simulink model "subsystem_118_bus_self_clearing_blocking"  (R2025b)
settings: Solver=ode45  StartTime=0.0  StopTime=Tstop  FixedStep=Ts  RelTol=1e-12  AbsTol=1e-12
values from neighbouring files (symbols this model uses):
  gfl3_enable_before = ones(numberOfGFLs,1)    [plotFun.m]
  gfl3_enable_blocked = gfl3_enable_before    [plotFun.m]
  gfl3_enable_clear_increment = gfl3_enable_before - gfl3_enable_blocked    [plotFun.m]
  gfl3_enable_zero = zeros(numberOfGFLs,1)    [plotFun.m]
  Imax = 15    [config_file.m]
  nominalInter =     [nominalInter.mat]
  nominalU =     [nominalU.mat]
  nominalY =     [nominalY.mat]
  P_input = 0    [main_sub_118_bus.m]    (also in plotFun.m = 0.03)
  sub = struct    [main_sub_118_bus.m]
  sys_j = sys_j(1:end-1)    [IBR_modelGenerator.m]
  sys_j_AA = sys_j    [modularMOR_main.m]
  sys_j_BT = sys_j    [modularMOR_main.m]
  Tclear_gfl = 0.11    [plotFun.m]
  Tstep_gfl = 0.1    [main_sub_118_bus.m]
  Tstep_gfm = 0.1    [main_sub_118_bus.m]
  Ttrip_gfl = 0.1    [plotFun.m]
  w = 2*pi*50    (= 314.159265359)    [config_file.m]    (also in mirrorMimoWeightedFrequencyData.m = w(:); modularMOR_main.m = w(:).'; plotTest.m = w(:).')
undefined symbols (not defined in the file or in its folder): con_sub, linSys1, linSys2, linSys3
libraries: simulink x10
(part 5 of 7)

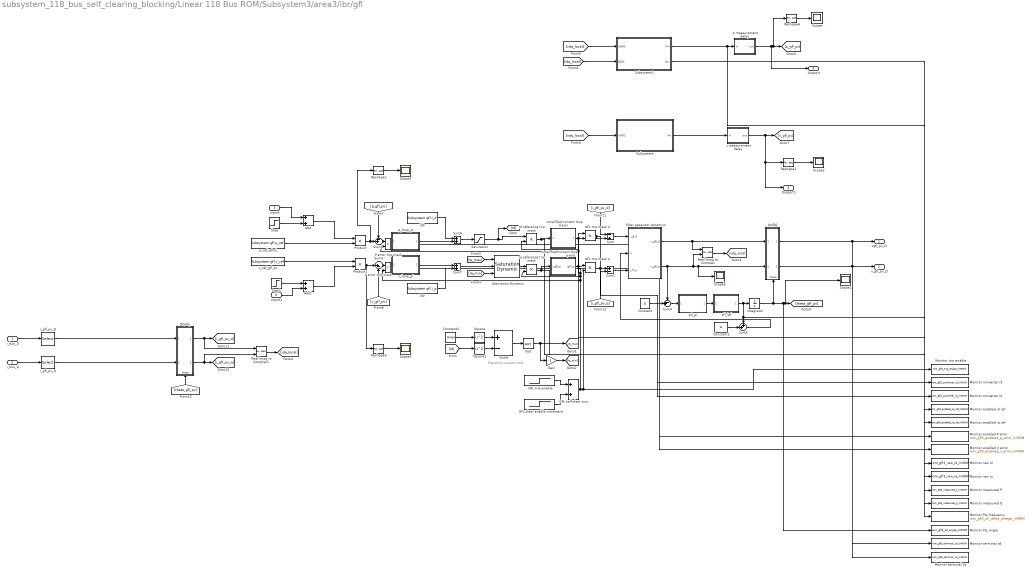
== system subsystem_118_bus_self_clearing_blocking/Linear 118 Bus ROM/Subsystem3/area3/ibr/gfl ==
  note: P-priority current limit
  i_bus_D : Inport
  i_bus_Q : Inport  Port=2
  Inport : Inport  Port=3
  Inport1 : Inport  Port=4
  Add : Sum
  Add1 : Sum
  Constant : Constant  Value=0
  Constant1 : Constant  Value=w
  Constant2 : Constant  Value=Imax
  DQ/dq : Subsystem
      settings: PortSchema="{\"entries\":[{\"content\":{\"sides\":[{\"content\":{\"connectorIds\":[\"In1\",\"In2\"]},\"type\":\"ConnectorPlacement.EquallySpacedRectSide\",\"uuid\":\"6aba5a73-e9d3-440a-9da8-5b4060b79a22\"},{\"content\":{\"connectorIds\":[\"Out1\",\"Out2\"],\"side\":\"RIGHT\"},\"type\":\"ConnectorPlacement.EquallySpacedRectSide\",\"uuid\":\"fb100e33-0f2b-446b-b234-6a01cff1cf94\"},{\"content\":{\"connectorIds\":[],\"side\":\"TOP\"},\"type\":\"ConnectorPlacement.EquallySpacedRectSide\",\"uuid\":\"cb346bab-8363-4920-b8bd-1af08716b150\"},{\"content\":{\"connectorIds\":[\"In3\"],\"side\":\"BOTTOM\"},\"type\":\"ConnectorPlacement.EquallySpacedRectSide\",\"uuid\":\"daf67601-a33f-44c6-bbbf-d32eadf086e5\"},{\"content\":{\"connectorIds\":[],\"side\":\"HIDDEN\"},\"type\":\"ConnectorPlacement.EquallySpacedRectSide\",\"uuid\":\"157b31a2-d1ec-4854-8b21-1495795af5ef\"}]},\"type\":\"ConnectorPlacement.EquallySpacedConnector\",\"uuid\":\"bdcd0df2-60ef-4202-9e13-560935cf5e64\"}],\"packageUris\":[\"http://schema.mathworks.com/mf0/Connector/R2020b\"],\"version\":\"1.0\"}"
      mask Display: image('$imagefile'); % Use "Edit Image" on toolstrip to change.
  GFL clear enable increment : Step  Time=Tclear_gfl  Before=gfl3_enable_zero  After=gfl3_enable_clear_increment  SampleTime=0
  GFL self-clear sum : Sum
  GFL trip enable : Step  Time=Ttrip_gfl  Before=gfl3_enable_before  After=gfl3_enable_blocked  SampleTime=0
  GFL trip mask d : Product  Inputs=**
  GFL trip mask q : Product  Inputs=**
  Gain : Gain  Gain=-1
  Id reference trip mask : Product  Inputs=**
  Integrator : Integrator  InitialCondition=Subsystem.gfl.theta  ContinuousStateAttributes='gfl_osc'
  Iq reference trip mask : Product  Inputs=**
  Monitor PLL angle : ToWorkspace  VariableName=rom_gfl3_pll_angle_linROM  SaveFormat=Timeseries  SampleTime=-1
  Monitor PLL frequency : ToWorkspace  VariableName=rom_gfl3_pll_delta_omega_linROM  SaveFormat=Timeseries  SampleTime=-1
  Monitor converter id : ToWorkspace  VariableName=rom_gfl3_converter_id_linROM  SaveFormat=Timeseries  SampleTime=-1
  Monitor converter iq : ToWorkspace  VariableName=rom_gfl3_converter_iq_linROM  SaveFormat=Timeseries  SampleTime=-1
  Monitor enabled P error : ToWorkspace  VariableName=rom_gfl3_enabled_p_error_linROM  SaveFormat=Timeseries  SampleTime=-1
  Monitor enabled V error : ToWorkspace  VariableName=rom_gfl3_enabled_v_error_linROM  SaveFormat=Timeseries  SampleTime=-1
  Monitor enabled id ref : ToWorkspace  VariableName=rom_gfl3_enabled_id_ref_linROM  SaveFormat=Timeseries  SampleTime=-1
  Monitor enabled iq ref : ToWorkspace  VariableName=rom_gfl3_enabled_iq_ref_linROM  SaveFormat=Timeseries  SampleTime=-1
  Monitor measured P : ToWorkspace  VariableName=rom_gfl3_measured_p_linROM  SaveFormat=Timeseries  SampleTime=-1
  Monitor measured Q : ToWorkspace  VariableName=rom_gfl3_measured_q_linROM  SaveFormat=Timeseries  SampleTime=-1
  Monitor raw id : ToWorkspace  VariableName=rom_gfl3_raw_id_linROM  SaveFormat=Timeseries  SampleTime=-1
  Monitor raw iq : ToWorkspace  VariableName=rom_gfl3_raw_iq_linROM  SaveFormat=Timeseries  SampleTime=-1
  Monitor terminal vd : ToWorkspace  VariableName=rom_gfl3_terminal_vd_linROM  SaveFormat=Timeseries  SampleTime=-1
  Monitor terminal vq : ToWorkspace  VariableName=rom_gfl3_terminal_vq_linROM  SaveFormat=Timeseries  SampleTime=-1
  Monitor trip enable : ToWorkspace  VariableName=rom_gfl3_trip_enable_linROM  SaveFormat=Timeseries  SampleTime=-1
  P error trip mask : Product  Inputs=**
  Product : Product
  Product1 : Product
  Real-Imag to Complex : RealImagToComplex
  Real-Imag to Complex1 : RealImagToComplex
  Reshape{1..4} (4 alike) : Reshape
  Saturation : Saturate  UpperLimit=Imax  LowerLimit=-Imax
  Saturation Dynamic : simulink/Discontinuities/Saturation Dynamic  OutMin=[]  OutMax=[]  OutDataTypeStr=Inherit: Same as second input  OutDataType=fixdt(1, 16)  OutScaling=2^-10  DoSatur=off
  Scope{,1..5} (6 alike) : Scope
      Scope settings: ActiveDisplayYMinimum=-1  ActiveDisplayYMaximum=1  DataLoggingVariableName=pm_gfl  DataLoggingSaveFormat=Structure
      Scope1 settings: ActiveDisplayYMinimum=-0.38233203386380687  ActiveDisplayYMaximum=-0.24913479990794113  DataLoggingVariableName=thetagflwnd  DataLoggingSaveFormat=Structure
      Scope2 settings: ActiveDisplayYMinimum=-1  ActiveDisplayYMaximum=1  DataLoggingVariableName=vm_gfl  DataLoggingSaveFormat=Structure
      Scope3 settings: ActiveDisplayYMinimum=0.75  ActiveDisplayYMaximum=0.95  DataLoggingVariableName=pr_gfl  DataLoggingSaveFormat=Structure
      Scope4 settings: ActiveDisplayYMinimum=1.02188  ActiveDisplayYMaximum=1.05312  DataLoggingVariableName=vr_gfl  DataLoggingSaveFormat=Structure
      Scope5 settings: DataLoggingVariableName=ScopeData3
  Sqrt : Sqrt
  Square : Math  Operator=square
  Square1 : Math  Operator=square
  Step : Step  Time=Tstep_gfl  Before=Subsystem.P_before_gfl  After=Subsystem.P_after_gfl  SampleTime=0
  Step1 : Step  Time=Tstep_gfl  Before=Subsystem.V_before_gfl  After=Subsystem.V_after_gfl  SampleTime=0
  Subsystem : Subsystem
      mask Display: image('$imagefile'); % Use "Edit Image" on toolstrip to change.
  Subsystem1 : Subsystem
      mask Display: image('$imagefile'); % Use "Edit Image" on toolstrip to change.
  Sum : Sum  Inputs=-+
  Sum1 : Sum  Inputs=+-
  Sum2 : Sum  Inputs=-+|
  Sum3 : Sum  Inputs=|+-
  Sum4 : Sum  Inputs=-+|
  Sum5 : Sum  Inputs=++|
  Sum6 : Sum
  Sum7 : Sum
  Sum8 : Sum  Inputs=+-
  V error trip mask : Product  Inputs=**
  dq/DQ : Subsystem
      settings: PortSchema="{\"entries\":[{\"content\":{\"sides\":[{\"content\":{\"connectorIds\":[\"In1\",\"In2\"]},\"type\":\"ConnectorPlacement.EquallySpacedRectSide\",\"uuid\":\"6aba5a73-e9d3-440a-9da8-5b4060b79a22\"},{\"content\":{\"connectorIds\":[\"Out1\",\"Out2\"],\"side\":\"RIGHT\"},\"type\":\"ConnectorPlacement.EquallySpacedRectSide\",\"uuid\":\"fb100e33-0f2b-446b-b234-6a01cff1cf94\"},{\"content\":{\"connectorIds\":[],\"side\":\"TOP\"},\"type\":\"ConnectorPlacement.EquallySpacedRectSide\",\"uuid\":\"cb346bab-8363-4920-b8bd-1af08716b150\"},{\"content\":{\"connectorIds\":[\"In3\"],\"side\":\"BOTTOM\"},\"type\":\"ConnectorPlacement.EquallySpacedRectSide\",\"uuid\":\"daf67601-a33f-44c6-bbbf-d32eadf086e5\"},{\"content\":{\"connectorIds\":[],\"side\":\"HIDDEN\"},\"type\":\"ConnectorPlacement.EquallySpacedRectSide\",\"uuid\":\"157b31a2-d1ec-4854-8b21-1495795af5ef\"}]},\"type\":\"ConnectorPlacement.EquallySpacedConnector\",\"uuid\":\"bdcd0df2-60ef-4202-9e13-560935cf5e64\"}],\"packageUris\":[\"http://schema.mathworks.com/mf0/Connector/R2020b\"],\"version\":\"1.0\"}"
      mask Display: image('$imagefile'); % Use "Edit Image" on toolstrip to change.
  filter capacitor dynamics : Subsystem
      mask Display: image('$imagefile'); % Use "Edit Image" on toolstrip to change.
  i_gfl_pv_D : Selector  InputPortWidth=size(Subsystem.sys_data,1)  IndexOptions=Index vector (dialog)  Indices=Subsystem.busnum.gfl  OutputSizes=1
  i_gfl_pv_Q : Selector  InputPortWidth=size(Subsystem.sys_data,1)  IndexOptions=Index vector (dialog)  Indices=Subsystem.busnum.gfl  OutputSizes=1
  id0 : Constant  Value=Subsystem.gfl.i_d
  iq0 : Constant  Value=Subsystem.gfl.i_q
  p measurement delay : Subsystem
      mask Display: image('$imagefile'); % Use "Edit Image" on toolstrip to change.
  p_loop_pi : Subsystem
      mask Display: image('$imagefile'); % Use "Edit Image" on toolstrip to change.
  p_ref_gfm2 : Constant  Value=Subsystem.gfl.p_ref
  pll_lpf : Subsystem
      mask Display: image('$imagefile'); % Use "Edit Image" on toolstrip to change.
  pll_pi : Subsystem
      mask Display: image('$imagefile'); % Use "Edit Image" on toolstrip to change.
  simplified current loop d-axis : Subsystem
      mask Display: image('$imagefile'); % Use "Edit Image" on toolstrip to change.
  simplified current loop q-axis : Subsystem
      mask Display: image('$imagefile'); % Use "Edit Image" on toolstrip to change.
  v measurement delay : Subsystem
      mask Display: image('$imagefile'); % Use "Edit Image" on toolstrip to change.
  v_loop_pi : Subsystem
      mask Display: image('$imagefile'); % Use "Edit Image" on toolstrip to change.
  v_ref_gfl_pv : Constant  Value=Subsystem.gfl.v_ref
  vgfl_pv_D : Outport
  v_gfl_pv_Q : Outport  Port=2
  Outport : Outport  Port=3
  Outport1 : Outport  Port=4
  wires:
  pll_lpf/1(LPF_output) -> Monitor PLL frequency/1, Sum5/1, Integrator/1
  Constant/1 -> Sum4/2
  filter capacitor dynamics/1(v_gfl_d) -> dq/DQ/1(d-quantity), Real-Imag to Complex/1
  v measurement delay/1(out) -> Reshape1/1, Outport1/1, [v_gfl_pv]
  filter capacitor dynamics/2(v_gfl_q) -> Real-Imag to Complex/2, Scope5/1, dq/DQ/2(q-quantity), Sum4/1
  [p_gfl_pv] -> Sum2/1
  Sum1/1 -> filter capacitor dynamics/3(i_cf_q)
  Sum4/1 -> pll_pi/1("  ")
  Sum5/1 -> filter capacitor dynamics/2(w)
  dq/DQ/1(D-quantity) -> vgfl_pv_D/1, Monitor terminal vd/1
  p measurement delay/1(out) -> Outport/1, Reshape4/1, [p_gfl_pv]
  Constant1/1 -> Sum5/2
  [i_gfl_pv_d] -> Sum/1
  Sum/1 -> filter capacitor dynamics/1(i_cf_d)
  [i_gfl_pv_q] -> Sum1/2
  [theta_gfl_pv] -> DQ/dq/3(theta)
  pll_pi/1(" ") -> pll_lpf/1(LPF_input)
  [v_gfl_pv] -> Sum3/2
  i_bus_Q/1 -> i_gfl_pv_Q/1
  i_bus_D/1 -> i_gfl_pv_D/1
  p_loop_pi/1(" ") -> Sum6/2
  v_loop_pi/1(" ") -> Sum7/1
  iq0/1 -> Sum7/2
  id0/1 -> Sum6/1
  Sum6/1 -> Saturation/1
  Integrator/1 -> Monitor PLL angle/1, Scope1/1, [theta_gfl_pv], dq/DQ/3(theta)
  Reshape4/1 -> Scope/1
  Reshape1/1 -> Scope2/1
  [Id] -> Square1/1
  Gain/1 -> [Iq_min]
  Constant2/1 -> Square/1
  Square/1 -> Sum8/1
  Sqrt/1 -> [Iq_max], Gain/1
  Square1/1 -> Sum8/2
  Sum8/1 -> Sqrt/1
  Saturation/1 -> [Id], Id reference trip mask/1
  Sum7/1 -> Saturation Dynamic/2
  [Iq_max] -> Saturation Dynamic/1
  [Iq_min] -> Saturation Dynamic/3
  [vdq_local] -> Subsystem/1(vbDQ)
  [vdq_local] -> Subsystem1/1(vbDQ)
  [idq_local] -> Subsystem1/2(IbDQ)
  Real-Imag to Complex/1 -> [vdq_local]
  DQ/dq/1(d_quantity) -> Real-Imag to Complex1/1, [i_gfl_pv_d]
  DQ/dq/2(q_quantity) -> Real-Imag to Complex1/2, [i_gfl_pv_q]
  Real-Imag to Complex1/1 -> [idq_local]
  dq/DQ/2(Q-quantity) -> v_gfl_pv_Q/1, Monitor terminal vq/1
  Subsystem/1(Vm) -> v measurement delay/1(in)
  Subsystem1/1(Pm) -> p measurement delay/1(in), Monitor measured P/1
  p_ref_gfm2/1 -> Product/2
  v_ref_gfl_pv/1 -> Product1/1
  Reshape2/1 -> Scope3/1
  Product/1 -> Reshape2/1, Sum2/2
  Reshape3/1 -> Scope4/1
  Product1/1 -> Sum3/1, Reshape3/1
  Step/1 -> Add/2
  Add/1 -> Product/1
  Step1/1 -> Add1/1
  Add1/1 -> Product1/2
  Inport/1 -> Add/1
  Inport1/1 -> Add1/2
  i_gfl_pv_D/1 -> DQ/dq/1(D_quantity)
  i_gfl_pv_Q/1 -> DQ/dq/2(Q_quantity)
  simplified current loop d-axis/1("  ") -> GFL trip mask d/1, Monitor raw id/1
  GFL trip mask d/1 -> Sum/2, Monitor converter id/1
  simplified current loop q-axis/1(igfl_q) -> GFL trip mask q/1, Monitor raw iq/1
  GFL trip mask q/1 -> Sum1/1, Monitor converter iq/1
  Id reference trip mask/1 -> simplified current loop d-axis/1(" "), Monitor enabled id ref/1
  Saturation Dynamic/1 -> Iq reference trip mask/1
  Iq reference trip mask/1 -> simplified current loop q-axis/1(i_gfl_q), Monitor enabled iq ref/1
  Sum2/1 -> P error trip mask/1
  P error trip mask/1 -> p_loop_pi/1("  "), Monitor enabled P error/1
  Sum3/1 -> V error trip mask/1
  V error trip mask/1 -> v_loop_pi/1("  "), Monitor enabled V error/1
  Subsystem1/2(Qm) -> Monitor measured Q/1
  GFL trip enable/1 -> GFL self-clear sum/1
  GFL clear enable increment/1 -> GFL self-clear sum/2
  GFL self-clear sum/1 -> GFL trip mask q/2, Monitor trip enable/1, P error trip mask/2, Id reference trip mask/2, GFL trip mask d/2, Iq reference trip mask/2, V error trip mask/2

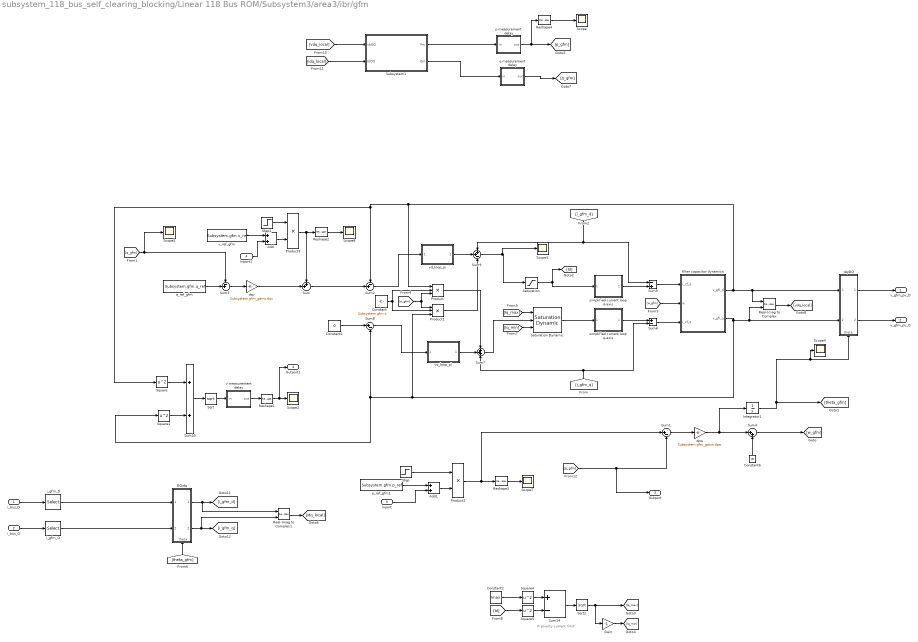
== system subsystem_118_bus_self_clearing_blocking/Linear 118 Bus ROM/Subsystem3/area3/ibr/gfm ==
  note: P-priority current limit
  i_bus_D : Inport
  i_bus_Q : Inport  Port=2
  Inport : Inport  Port=3
  Inport1 : Inport  Port=4
  Add : Sum
  Add1 : Sum
  Constant : Constant  Value=Subsystem.gfm.c
  Constant1 : Constant  Value=0
  Constant2 : Constant  Value=Imax
  Constant6 : Constant  Value=w
  DQ/dq : Subsystem
      settings: PortSchema="{\"entries\":[{\"content\":{\"sides\":[{\"content\":{\"connectorIds\":[\"In1\",\"In2\"]},\"type\":\"ConnectorPlacement.EquallySpacedRectSide\",\"uuid\":\"6aba5a73-e9d3-440a-9da8-5b4060b79a22\"},{\"content\":{\"connectorIds\":[\"Out1\",\"Out2\"],\"side\":\"RIGHT\"},\"type\":\"ConnectorPlacement.EquallySpacedRectSide\",\"uuid\":\"fb100e33-0f2b-446b-b234-6a01cff1cf94\"},{\"content\":{\"connectorIds\":[],\"side\":\"TOP\"},\"type\":\"ConnectorPlacement.EquallySpacedRectSide\",\"uuid\":\"cb346bab-8363-4920-b8bd-1af08716b150\"},{\"content\":{\"connectorIds\":[\"In3\"],\"side\":\"BOTTOM\"},\"type\":\"ConnectorPlacement.EquallySpacedRectSide\",\"uuid\":\"daf67601-a33f-44c6-bbbf-d32eadf086e5\"},{\"content\":{\"connectorIds\":[],\"side\":\"HIDDEN\"},\"type\":\"ConnectorPlacement.EquallySpacedRectSide\",\"uuid\":\"157b31a2-d1ec-4854-8b21-1495795af5ef\"}]},\"type\":\"ConnectorPlacement.EquallySpacedConnector\",\"uuid\":\"bdcd0df2-60ef-4202-9e13-560935cf5e64\"}],\"packageUris\":[\"http://schema.mathworks.com/mf0/Connector/R2020b\"],\"version\":\"1.0\"}"
      mask Display: image('$imagefile'); % Use "Edit Image" on toolstrip to change.
  Gain : Gain  Gain=-1
  Integrator1 : Integrator  InitialCondition=Subsystem.gfm.theta  ContinuousStateAttributes='gfm_osc'
  Product : Product  Inputs=3
  Product1 : Product  Inputs=3
  Product2 : Product
  Product3 : Product
  Real-Imag to Complex : RealImagToComplex
  Real-Imag to Complex1 : RealImagToComplex
  Reshape{1..4} (4 alike) : Reshape
  Saturation : Saturate  UpperLimit=Imax  LowerLimit=-Imax
  Saturation Dynamic : simulink/Discontinuities/Saturation Dynamic  OutMin=[]  OutMax=[]  OutDataTypeStr=Inherit: Same as second input  OutDataType=fixdt(1, 16)  OutScaling=2^-10  DoSatur=off
  Scope{,1..2,4..5,7..8} (7 alike) : Scope
      Scope settings: ActiveDisplayYMinimum=-1  ActiveDisplayYMaximum=1  DataLoggingVariableName=pm_gfm  DataLoggingSaveFormat=Structure
      Scope1 settings: ActiveDisplayYMinimum=0.57567  ActiveDisplayYMaximum=1.70344
      Scope2 settings: ActiveDisplayYMinimum=1.02215  ActiveDisplayYMaximum=1.04295  DataLoggingVariableName=vm_gfm  DataLoggingSaveFormat=Structure
      Scope4 settings: ActiveDisplayYMinimum=-1  ActiveDisplayYMaximum=1  DataLoggingVariableName=thetagfmwnd  DataLoggingSaveFormat=Structure
      Scope5 settings: ActiveDisplayYMinimum=0.85975274896238685  ActiveDisplayYMaximum=1.0032219511840634  DataLoggingVariableName=qgfmwnd  DataLoggingSaveFormat=Structure
      Scope7 settings: ActiveDisplayYMinimum=-1  ActiveDisplayYMaximum=1  DataLoggingVariableName=pr_gfm  DataLoggingSaveFormat=Structure
      Scope8 settings: ActiveDisplayYMinimum=0.040000000000000036  ActiveDisplayYMaximum=2.04  DataLoggingVariableName=vr_gfm  DataLoggingSaveFormat=Structure
  Sqrt : Sqrt
  Sqrt2 : Sqrt
  Square{,1,4..5} (4 alike) : Math  Operator=square
  Step : Step  Time=Tstep_gfm  Before=Subsystem.P_before_gfm  After=Subsystem.P_after_gfm
  Step1 : Step  Time=Tstep_gfm  Before=Subsystem.V_before_gfm  After=Subsystem.V_after_gfm
  Subsystem1 : Subsystem
      mask Display: image('$imagefile'); % Use "Edit Image" on toolstrip to change.
  Sum : Sum  Inputs=++|
  Sum1 : Sum  Inputs=|+-
  Sum10 : Sum
  Sum14 : Sum  Inputs=+-
  Sum2 : Sum  Inputs=-+|
  Sum3 : Sum  Inputs=-+|
  Sum4 : Sum  Inputs=|++
  Sum5 : Sum  Inputs=-+
  Sum6 : Sum  Inputs=+-
  Sum7 : Sum  Inputs=+++
  Sum8 : Sum  Inputs=|+-
  Sum9 : Sum  Inputs=++-
  dpw : Gain  Gain=Subsystem.gfm_gains.dpw
  dq/DQ : Subsystem
      settings: PortSchema="{\"entries\":[{\"content\":{\"sides\":[{\"content\":{\"connectorIds\":[\"In1\",\"In2\"]},\"type\":\"ConnectorPlacement.EquallySpacedRectSide\",\"uuid\":\"6aba5a73-e9d3-440a-9da8-5b4060b79a22\"},{\"content\":{\"connectorIds\":[\"Out1\",\"Out2\"],\"side\":\"RIGHT\"},\"type\":\"ConnectorPlacement.EquallySpacedRectSide\",\"uuid\":\"fb100e33-0f2b-446b-b234-6a01cff1cf94\"},{\"content\":{\"connectorIds\":[],\"side\":\"TOP\"},\"type\":\"ConnectorPlacement.EquallySpacedRectSide\",\"uuid\":\"cb346bab-8363-4920-b8bd-1af08716b150\"},{\"content\":{\"connectorIds\":[\"In3\"],\"side\":\"BOTTOM\"},\"type\":\"ConnectorPlacement.EquallySpacedRectSide\",\"uuid\":\"daf67601-a33f-44c6-bbbf-d32eadf086e5\"},{\"content\":{\"connectorIds\":[],\"side\":\"HIDDEN\"},\"type\":\"ConnectorPlacement.EquallySpacedRectSide\",\"uuid\":\"157b31a2-d1ec-4854-8b21-1495795af5ef\"}]},\"type\":\"ConnectorPlacement.EquallySpacedConnector\",\"uuid\":\"bdcd0df2-60ef-4202-9e13-560935cf5e64\"}],\"packageUris\":[\"http://schema.mathworks.com/mf0/Connector/R2020b\"],\"version\":\"1.0\"}"
      mask Display: image('$imagefile'); % Use "Edit Image" on toolstrip to change.
  dqv : Gain  Gain=Subsystem.gfm_gains.dqv
  filter capacitor dynamics : Subsystem
      mask Display: image('$imagefile'); % Use "Edit Image" on toolstrip to change.
  i_gfm_D : Selector  InputPortWidth=size(Subsystem.sys_data,1)  IndexOptions=Index vector (dialog)  Indices=Subsystem.busnum.gfm  OutputSizes=1
  i_gfm_Q : Selector  InputPortWidth=size(Subsystem.sys_data,1)  IndexOptions=Index vector (dialog)  Indices=Subsystem.busnum.gfm  OutputSizes=1
  p measurement delay : Subsystem
      mask Display: image('$imagefile'); % Use "Edit Image" on toolstrip to change.
  p_ref_gfm1 : Constant  Value=Subsystem.gfm.p_ref
  q measurement delay : Subsystem
      mask Display: image('$imagefile'); % Use "Edit Image" on toolstrip to change.
  q_ref_gfm : Constant  Value=Subsystem.gfm.q_ref
  simplified current loop d-axis : Subsystem
      mask Display: image('$imagefile'); % Use "Edit Image" on toolstrip to change.
  simplified current loop q-axis : Subsystem
      mask Display: image('$imagefile'); % Use "Edit Image" on toolstrip to change.
  v measurement delay : Subsystem
      mask Display: image('$imagefile'); % Use "Edit Image" on toolstrip to change.
  v_ref_gfm : Constant  Value=Subsystem.gfm.v_ref
  vd_loop_pi : Subsystem
      mask Display: image('$imagefile'); % Use "Edit Image" on toolstrip to change.
  vq_loop_pi : Subsystem
      mask Display: image('$imagefile'); % Use "Edit Image" on toolstrip to change.
  v_gfm_pv_D : Outport
  v_gfm_pv_Q : Outport  Port=2
  Outport : Outport  Port=3
  Outport1 : Outport  Port=4
  wires:
  Sum2/1 -> vd_loop_pi/1("  ")
  dq/DQ/1(D-quantity) -> v_gfm_pv_D/1
  dq/DQ/2(Q-quantity) -> v_gfm_pv_Q/1
  dpw/1 -> Sum4/1, Integrator1/1
  [p_gfm] -> Outport/1, Sum1/2
  Constant6/1 -> Sum4/2
  Sum1/1 -> dpw/1
  Integrator1/1 -> [theta_gfm], Scope4/1, dq/DQ/3(theta)
  Sum/1 -> Sum2/2
  dqv/1 -> Sum/2
  Sum3/1 -> dqv/1
  q_ref_gfm/1 -> Sum3/2
  [q_gfm] -> Sum3/1, Scope5/1
  Sum6/1 -> filter capacitor dynamics/3(i_cf_q)
  simplified current loop q-axis/1("  ") -> Sum6/1
  Sum5/1 -> filter capacitor dynamics/1(i_cf_d)
  [theta_gfm] -> DQ/dq/3(theta)
  vq_loop_pi/1(" ") -> Sum7/2
  Sum8/1 -> vq_loop_pi/1("  ")
  vd_loop_pi/1(" ") -> Sum9/2
  [i_gfm_q] -> Sum6/2, Sum7/3
  [i_gfm_d] -> Sum5/1, Sum9/1
  Product/1 -> Sum7/1
  Product1/1 -> Sum9/3
  Sum4/1 -> [w_gfm]
  [w_gfm] -> filter capacitor dynamics/2(w)
  [w_gfm] -> Product/3, Product1/1
  Constant/1 -> Product1/2, Product/2
  Constant1/1 -> Sum8/1
  simplified current loop d-axis/1("  ") -> Sum5/2
  Square/1 -> Sum10/1
  Square1/1 -> Sum10/2
  Sum10/1 -> Sqrt/1
  Sqrt/1 -> v measurement delay/1(in)
  v measurement delay/1(out) -> Reshape1/1
  Product2/1 -> Sum1/1, Reshape3/1
  Step/1 -> Product2/1
  Step1/1 -> Product3/1
  Product3/1 -> Reshape2/1, Sum/1
  Sum7/1 -> Saturation Dynamic/2
  [Iq_max] -> Saturation Dynamic/1
  [Iq_min] -> Saturation Dynamic/3
  Saturation/1 -> simplified current loop d-axis/1(" "), [Id]
  Saturation Dynamic/1 -> simplified current loop q-axis/1(" ")
  Sum9/1 -> Scope1/1, Saturation/1
  Square5/1 -> Sum14/2
  Sum14/1 -> Sqrt2/1
  Sqrt2/1 -> [Iq_max], Gain/1
  Constant2/1 -> Square4/1
  Gain/1 -> [Iq_min]
  Square4/1 -> Sum14/1
  [Id] -> Square5/1
  i_bus_Q/1 -> i_gfm_Q/1
  i_bus_D/1 -> i_gfm_D/1
  i_gfm_D/1 -> DQ/dq/1(D_quantity)
  i_gfm_Q/1 -> DQ/dq/2(Q_quantity)
  Subsystem1/1(Pm) -> p measurement delay/1(in)
  Reshape4/1 -> Scope/1
  p measurement delay/1(out) -> [p_gfm], Reshape4/1
  [vdq_local] -> Subsystem1/1(vbDQ)
  [idq_local] -> Subsystem1/2(IbDQ)
  Real-Imag to Complex1/1 -> [idq_local]
  DQ/dq/2(q_quantity) -> Real-Imag to Complex1/2, [i_gfm_q]
  DQ/dq/1(d_quantity) -> Real-Imag to Complex1/1, [i_gfm_d]
  filter capacitor dynamics/2(v_gfl_q) -> Real-Imag to Complex/2, dq/DQ/2(q-quantity), Product1/3, Square1/1, Sum8/2
  Real-Imag to Complex/1 -> [vdq_local]
  filter capacitor dynamics/1(v_gfl_d) -> Real-Imag to Complex/1, dq/DQ/1(d-quantity), Product/1, Sum2/1, Square/1
  Subsystem1/2(Qm) -> q measurement delay/1(in)
  q measurement delay/1(out) -> [q_gfm]
  Reshape2/1 -> Scope8/1
  Reshape3/1 -> Scope7/1
  Reshape1/1 -> Outport1/1, Scope2/1
  Add/1 -> Product3/2
  v_ref_gfm/1 -> Add/1
  Add1/1 -> Product2/2
  p_ref_gfm1/1 -> Add1/1
  Inport/1 -> Add1/2
  Inport1/1 -> Add/2

== system subsystem_118_bus_self_clearing_blocking/Linear 118 Bus ROM/Subsystem3/area3/non_ibr/floating buses ==
  In1 : Inport
  In2 : Inport  Port=2
  i_float_D : Selector  InputPortWidth=size(Subsystem.sys_data,1)  IndexOptions=Index vector (dialog)  Indices=Subsystem.busnum.float  OutputSizes=1
  i_float_Q : Selector  InputPortWidth=size(Subsystem.sys_data,1)  IndexOptions=Index vector (dialog)  Indices=Subsystem.busnum.float  OutputSizes=1
  line charging dynamics : Subsystem
      mask Display: image('$imagefile'); % Use "Edit Image" on toolstrip to change.
  v_float_D : Outport
  v_float_Q : Outport  Port=2
  wires:
  i_float_D/1 -> line charging dynamics/1(i_float_D)
  In2/1 -> i_float_Q/1
  i_float_Q/1 -> line charging dynamics/2(i_float_Q)
  In1/1 -> i_float_D/1
  line charging dynamics/2(v_float_Q) -> v_float_Q/1
  line charging dynamics/1(v_float_D) -> v_float_D/1

== system subsystem_118_bus_self_clearing_blocking/Linear 118 Bus ROM/Subsystem3/area3/non_ibr/infinite bus ==
  v_inf_D : Constant  Value=Subsystem.infbus.v_D
  v_inf_Q : Constant  Value=Subsystem.infbus.v_Q
  Out1 : Outport
  Out2 : Outport  Port=2
  wires:
  v_inf_Q/1 -> Out2/1
  v_inf_D/1 -> Out1/1

== system subsystem_118_bus_self_clearing_blocking/Linear 118 Bus ROM/Subsystem3/area3/non_ibr/load buses ==
  In1 : Inport
  In2 : Inport  Port=2
  Constant : Constant  Value=Subsystem.load1.v_D
  Constant1 : Constant  Value=Subsystem.load1.v_Q
  Constant2 : Constant  Value=Subsystem.load1.ptype
  Constant3 : Constant  Value=Subsystem.load1.qtype
  Divide : Product  Inputs=*/
  Product : Product
  Product1 : Product
  Sqrt : Sqrt
  Sqrt1 : Sqrt
  Square1 : Math  Operator=pow
  Square{2..5} (4 alike) : Math  Operator=square
  Square6 : Math  Operator=pow
  Subsystem : Subsystem
  Sum : Sum  Inputs=|-+
  Sum1 : Sum  Inputs=|-+
  Sum2 : Sum
  Sum4 : Sum
  i_load_D : Selector  InputPortWidth=size(Subsystem.sys_data,1)  IndexOptions=Index vector (dialog)  Indices=Subsystem.busnum.load  OutputSizes=1
  i_load_Q : Selector  InputPortWidth=size(Subsystem.sys_data,1)  IndexOptions=Index vector (dialog)  Indices=Subsystem.busnum.load  OutputSizes=1
  line charging dynamics : Subsystem
      mask Display: image('$imagefile'); % Use "Edit Image" on toolstrip to change.
  load bus p : Constant  Value=Subsystem.load1.p
  load bus q : Constant  Value=Subsystem.load1.q
  Out1 : Outport
  Out2 : Outport  Port=2
  wires:
  In1/1 -> i_load_D/1
  In2/1 -> i_load_Q/1
  Sum1/1 -> line charging dynamics/2(i_load_c_Q)
  i_load_Q/1 -> Sum1/1
  i_load_D/1 -> Sum/1
  [v_load_D] -> Subsystem/3(vD)
  [v_load_Q] -> Subsystem/4(vQ)
  Subsystem/2(i_inj_load_q) -> Sum1/2
  Subsystem/1(i_inj_load_d) -> Sum/2
  Sum/1 -> line charging dynamics/1(i_load_c_D)
  load bus p/1 -> Product/1
  Square6/1 -> Product/2
  Product/1 -> Subsystem/1(p)
  Product1/1 -> Subsystem/2(q)
  load bus q/1 -> Product1/2
  line charging dynamics/1(v_load_D) -> Out1/1, [v_load_D]
  line charging dynamics/2(v_load_Q) -> Out2/1, [v_load_Q]
  Square1/1 -> Product1/1
  Sum2/1 -> Sqrt1/1
  Square4/1 -> Sum2/1
  Constant1/1 -> Square3/1
  [v_load_D] -> Square4/1
  Square5/1 -> Sum2/2
  Constant2/1 -> Square6/2
  Divide/1 -> Square6/1, Square1/1
  Constant/1 -> Square2/1
  Sqrt/1 -> Divide/2
  Square3/1 -> Sum4/2
  Sqrt1/1 -> Divide/1
  Sum4/1 -> Sqrt/1
  Square2/1 -> Sum4/1
  [v_load_Q] -> Square5/1
  Constant3/1 -> Square1/2

== system subsystem_118_bus_self_clearing_blocking/Subsystem1/area1/ibr/gfl/DQ//dq ==
  D_quantity : Inport
  Q_quantity : Inport  Port=2
  theta : Inport  Port=3
  Complex to Magnitude-Angle : ComplexToMagnitudeAngle
  Complex to Real-Imag : ComplexToRealImag
  Magnitude-Angle to Complex : MagnitudeAngleToComplex
  Real-Imag to Complex : RealImagToComplex
  Sum : Sum  Inputs=|+-
  d_quantity : Outport
  q_quantity : Outport  Port=2
  wires:
  D_quantity/1 -> Real-Imag to Complex/1
  Complex to Magnitude-Angle/2 -> Sum/1
  Complex to Magnitude-Angle/1 -> Magnitude-Angle to Complex/1
  Real-Imag to Complex/1 -> Complex to Magnitude-Angle/1
  Sum/1 -> Magnitude-Angle to Complex/2
  Q_quantity/1 -> Real-Imag to Complex/2
  Magnitude-Angle to Complex/1 -> Complex to Real-Imag/1
  Complex to Real-Imag/1 -> d_quantity/1
  Complex to Real-Imag/2 -> q_quantity/1
  theta/1 -> Sum/2

== system subsystem_118_bus_self_clearing_blocking/Subsystem1/area1/ibr/gfl/Subsystem ==
  vbDQ : Inport
  Abs : Abs  SaturateOnIntegerOverflow=off
  Vm : Outport
  wires:
  Abs/1 -> Vm/1
  vbDQ/1 -> Abs/1

== system subsystem_118_bus_self_clearing_blocking/Subsystem1/area1/ibr/gfl/Subsystem1 ==
  vbDQ : Inport
  IbDQ : Inport  Port=2
  Complex to Real-Imag : ComplexToRealImag
  Complex to Real-Imag1 : ComplexToRealImag
  Product{,1..3} (4 alike) : Product
  Sum : Sum
  Sum1 : Sum  Inputs=+-
  Pm : Outport
  Qm : Outport  Port=2
  wires:
  Product/1 -> Sum/1
  Product1/1 -> Sum/2
  Sum/1 -> Pm/1
  Sum1/1 -> Qm/1
  Product3/1 -> Sum1/2
  Product2/1 -> Sum1/1
  [vbQ] -> Product2/1
  [IbD] -> Product2/2
  [vbD] -> Product3/1
  [IbQ] -> Product3/2
  [vbD] -> Product/1
  [IbD] -> Product/2
  [IbQ] -> Product1/2
  [vbQ] -> Product1/1
  vbDQ/1 -> Complex to Real-Imag/1
  Complex to Real-Imag/1 -> [vbD]
  Complex to Real-Imag/2 -> [vbQ]
  IbDQ/1 -> Complex to Real-Imag1/1
  Complex to Real-Imag1/1 -> [IbD]
  Complex to Real-Imag1/2 -> [IbQ]

== system subsystem_118_bus_self_clearing_blocking/Subsystem1/area1/ibr/gfl/dq//DQ ==
  d-quantity : Inport
  q-quantity : Inport  Port=2
  theta : Inport  Port=3
  Complex to Magnitude-Angle : ComplexToMagnitudeAngle
  Complex to Real-Imag : ComplexToRealImag
  Magnitude-Angle to Complex : MagnitudeAngleToComplex
  Real-Imag to Complex : RealImagToComplex
  Sum : Sum  Inputs=|++
  D-quantity : Outport
  Q-quantity : Outport  Port=2
  wires:
  d-quantity/1 -> Real-Imag to Complex/1
  Complex to Magnitude-Angle/2 -> Sum/1
  Complex to Magnitude-Angle/1 -> Magnitude-Angle to Complex/1
  Real-Imag to Complex/1 -> Complex to Magnitude-Angle/1
  Sum/1 -> Magnitude-Angle to Complex/2
  q-quantity/1 -> Real-Imag to Complex/2
  Magnitude-Angle to Complex/1 -> Complex to Real-Imag/1
  Complex to Real-Imag/1 -> D-quantity/1
  Complex to Real-Imag/2 -> Q-quantity/1
  theta/1 -> Sum/2

== system subsystem_118_bus_self_clearing_blocking/Subsystem1/area1/ibr/gfl/filter capacitor dynamics ==
  i_cf_d : Inport
  w : Inport  Port=2
  i_cf_q : Inport  Port=3
  1/C_gfl_pv : Gain  Gain=1./Subsystem.gfl.c
  "1/C_gfl_pv " : Gain  Gain=1./Subsystem.gfl.c
  Integrator : Integrator  InitialCondition=Subsystem.gfl.v_d  ContinuousStateAttributes='gfl_vd'
  Integrator1 : Integrator  InitialCondition=Subsystem.gfl.v_q  ContinuousStateAttributes='gfl_vq'
  Product : Product
  Product1 : Product
  Sum2 : Sum  Inputs=+-
  Sum3 : Sum
  v_gfl_d : Outport
  v_gfl_q : Outport  Port=2
  wires:
  w/1 -> [ws]
  [ws] -> Product/1
  Integrator/1 -> Product1/1, v_gfl_d/1
  Integrator1/1 -> Product/2, v_gfl_q/1
  [ws] -> Product1/2
  Sum3/1 -> Integrator/1
  Sum2/1 -> Integrator1/1
  1/C_gfl_pv/1 -> Sum3/2
  Product/1 -> Sum3/1
  "1/C_gfl_pv "/1 -> Sum2/1
  Product1/1 -> Sum2/2
  i_cf_d/1 -> 1/C_gfl_pv/1
  i_cf_q/1 -> "1/C_gfl_pv "/1

== system subsystem_118_bus_self_clearing_blocking/Subsystem1/area1/ibr/gfl/p measurement delay ==
  in : Inport
  Integrator1 : Integrator  InitialCondition=Subsystem.gfl.p_ref  ContinuousStateAttributes='gfl_p_m'
  Sum2 : Sum  Inputs=-+
  p_meas_bw : Gain  Gain=Subsystem.gfl.p_meas_w
  out : Outport
  wires:
  in/1 -> Sum2/2
  Sum2/1 -> p_meas_bw/1
  Integrator1/1 -> Sum2/1, out/1
  p_meas_bw/1 -> Integrator1/1

== system subsystem_118_bus_self_clearing_blocking/Subsystem1/area1/ibr/gfl/p_loop_pi ==
  "  " : Inport
  Integrator : Integrator  ContinuousStateAttributes='gfl_p_ctrl'
  Ki : Gain  Gain=Subsystem.gfl_gains.kip
  Kp : Gain  Gain=Subsystem.gfl_gains.kpp
  Sum : Sum  Inputs=|++
  " " : Outport
  wires:
  Kp/1 -> Sum/1
  Integrator/1 -> Sum/2
  Ki/1 -> Integrator/1
  "  "/1 -> Ki/1, Kp/1
  Sum/1 -> " "/1

== system subsystem_118_bus_self_clearing_blocking/Subsystem1/area1/ibr/gfl/pll_lpf ==
  LPF_input : Inport
  Integrator1 : Integrator  ContinuousStateAttributes='gfl_pll_lpf'
  Sum2 : Sum  Inputs=-+
  pll_lpf_bw : Gain  Gain=Subsystem.gfl.pll_lpf_w
  LPF_output : Outport
  wires:
  pll_lpf_bw/1 -> Integrator1/1
  Integrator1/1 -> LPF_output/1, Sum2/1
  Sum2/1 -> pll_lpf_bw/1
  LPF_input/1 -> Sum2/2

== system subsystem_118_bus_self_clearing_blocking/Subsystem1/area1/ibr/gfl/pll_pi ==
  "  " : Inport
  Integrator : Integrator  ContinuousStateAttributes='gfl_pll'
  Ki : Gain  Gain=Subsystem.gfl_gains.kipll
  Kp : Gain  Gain=Subsystem.gfl_gains.kppll
  Sum : Sum  Inputs=|++
  " " : Outport
  wires:
  Kp/1 -> Sum/1
  Integrator/1 -> Sum/2
  Ki/1 -> Integrator/1
  "  "/1 -> Ki/1, Kp/1
  Sum/1 -> " "/1

== system subsystem_118_bus_self_clearing_blocking/Subsystem1/area1/ibr/gfl/simplified current loop d-axis ==
  " " : Inport
  Gain : Gain  Gain=Subsystem.gfl.i_loop_w
  Integrator1 : Integrator  InitialCondition=Subsystem.gfl.i_d  ContinuousStateAttributes='gfl_id_ctrl'
  Sum2 : Sum  Inputs=-+
  "  " : Outport
  wires:
  Gain/1 -> Integrator1/1
  Integrator1/1 -> "  "/1, Sum2/1
  Sum2/1 -> Gain/1
  " "/1 -> Sum2/2

== system subsystem_118_bus_self_clearing_blocking/Subsystem1/area1/ibr/gfl/simplified current loop q-axis ==
  i_gfl_q : Inport
  Gain : Gain  Gain=Subsystem.gfl.i_loop_w
  Integrator1 : Integrator  InitialCondition=Subsystem.gfl.i_q  ContinuousStateAttributes='gfl_iq_ctrl'
  Sum2 : Sum  Inputs=-+
  igfl_q : Outport
  wires:
  Gain/1 -> Integrator1/1
  Integrator1/1 -> igfl_q/1, Sum2/1
  Sum2/1 -> Gain/1
  i_gfl_q/1 -> Sum2/2

== system subsystem_118_bus_self_clearing_blocking/Subsystem1/area1/ibr/gfl/v measurement delay ==
  in : Inport
  Integrator1 : Integrator  InitialCondition=Subsystem.gfl.v_ref  ContinuousStateAttributes='gfl_v_m'
  Sum2 : Sum  Inputs=-+
  v_meas_bw : Gain  Gain=Subsystem.gfl.v_meas_w
  out : Outport
  wires:
  in/1 -> Sum2/2
  Sum2/1 -> v_meas_bw/1
  Integrator1/1 -> Sum2/1, out/1
  v_meas_bw/1 -> Integrator1/1

== system subsystem_118_bus_self_clearing_blocking/Subsystem1/area1/ibr/gfl/v_loop_pi ==
  "  " : Inport
  Integrator : Integrator  ContinuousStateAttributes='gfl_v_ctrl'
  Ki : Gain  Gain=Subsystem.gfl_gains.kiv
  Kp : Gain  Gain=Subsystem.gfl_gains.kpv
  Sum : Sum  Inputs=|++
  " " : Outport
  wires:
  Kp/1 -> Sum/1
  Integrator/1 -> Sum/2
  Ki/1 -> Integrator/1
  "  "/1 -> Ki/1, Kp/1
  Sum/1 -> " "/1

== system subsystem_118_bus_self_clearing_blocking/Subsystem1/area1/ibr/gfm/DQ//dq ==
  D_quantity : Inport
  Q_quantity : Inport  Port=2
  theta : Inport  Port=3
  Complex to Magnitude-Angle : ComplexToMagnitudeAngle
  Complex to Real-Imag : ComplexToRealImag
  Magnitude-Angle to Complex : MagnitudeAngleToComplex
  Real-Imag to Complex : RealImagToComplex
  Sum : Sum  Inputs=|+-
  d_quantity : Outport
  q_quantity : Outport  Port=2
  wires:
  D_quantity/1 -> Real-Imag to Complex/1
  Complex to Magnitude-Angle/2 -> Sum/1
  Complex to Magnitude-Angle/1 -> Magnitude-Angle to Complex/1
  Real-Imag to Complex/1 -> Complex to Magnitude-Angle/1
  Sum/1 -> Magnitude-Angle to Complex/2
  Q_quantity/1 -> Real-Imag to Complex/2
  Magnitude-Angle to Complex/1 -> Complex to Real-Imag/1
  Complex to Real-Imag/1 -> d_quantity/1
  Complex to Real-Imag/2 -> q_quantity/1
  theta/1 -> Sum/2

== system subsystem_118_bus_self_clearing_blocking/Subsystem1/area1/ibr/gfm/Subsystem1 ==
  vbDQ : Inport
  IbDQ : Inport  Port=2
  Complex to Real-Imag : ComplexToRealImag
  Complex to Real-Imag1 : ComplexToRealImag
  Product{,1..3} (4 alike) : Product
  Sum : Sum
  Sum1 : Sum  Inputs=+-
  Pm : Outport
  Qm : Outport  Port=2
  wires:
  Product/1 -> Sum/1
  Product1/1 -> Sum/2
  Sum/1 -> Pm/1
  Sum1/1 -> Qm/1
  Product3/1 -> Sum1/2
  Product2/1 -> Sum1/1
  [vbQ] -> Product2/1
  [IbD] -> Product2/2
  [vbD] -> Product3/1
  [IbQ] -> Product3/2
  [vbD] -> Product/1
  [IbD] -> Product/2
  [IbQ] -> Product1/2
  [vbQ] -> Product1/1
  vbDQ/1 -> Complex to Real-Imag/1
  Complex to Real-Imag/1 -> [vbD]
  Complex to Real-Imag/2 -> [vbQ]
  IbDQ/1 -> Complex to Real-Imag1/1
  Complex to Real-Imag1/1 -> [IbD]
  Complex to Real-Imag1/2 -> [IbQ]

== system subsystem_118_bus_self_clearing_blocking/Subsystem1/area1/ibr/gfm/dq//DQ ==
  d-quantity : Inport
  q-quantity : Inport  Port=2
  theta : Inport  Port=3
  Complex to Magnitude-Angle : ComplexToMagnitudeAngle
  Complex to Real-Imag : ComplexToRealImag
  Magnitude-Angle to Complex : MagnitudeAngleToComplex
  Real-Imag to Complex : RealImagToComplex
  Sum : Sum  Inputs=|++
  D-quantity : Outport
  Q-quantity : Outport  Port=2
  wires:
  d-quantity/1 -> Real-Imag to Complex/1
  Complex to Magnitude-Angle/2 -> Sum/1
  Complex to Magnitude-Angle/1 -> Magnitude-Angle to Complex/1
  Real-Imag to Complex/1 -> Complex to Magnitude-Angle/1
  Sum/1 -> Magnitude-Angle to Complex/2
  q-quantity/1 -> Real-Imag to Complex/2
  Magnitude-Angle to Complex/1 -> Complex to Real-Imag/1
  Complex to Real-Imag/1 -> D-quantity/1
  Complex to Real-Imag/2 -> Q-quantity/1
  theta/1 -> Sum/2

== system subsystem_118_bus_self_clearing_blocking/Subsystem1/area1/ibr/gfm/filter capacitor dynamics ==
  i_cf_d : Inport
  w : Inport  Port=2
  i_cf_q : Inport  Port=3
  1/C_gfm : Gain  Gain=1./Subsystem.gfm.c
  "1/C_gfm " : Gain  Gain=1./Subsystem.gfm.c
  Display : Display
  Integrator : Integrator  InitialCondition=Subsystem.gfm.v_d  ContinuousStateAttributes='gfm_vd'
  Integrator1 : Integrator  InitialCondition=Subsystem.gfm.v_q  ContinuousStateAttributes='gfm_vq'
  Product : Product
  Product1 : Product
  Sum2 : Sum  Inputs=+-
  Sum3 : Sum
  v_gfl_d : Outport
  v_gfl_q : Outport  Port=2
  wires:
  w/1 -> [ws]
  [ws] -> Product/1
  Integrator/1 -> Product1/1, v_gfl_d/1
  Integrator1/1 -> Product/2, v_gfl_q/1
  [ws] -> Product1/2
  Sum3/1 -> Display/1, Integrator/1
  Sum2/1 -> Integrator1/1
  1/C_gfm/1 -> Sum3/2
  Product/1 -> Sum3/1
  "1/C_gfm "/1 -> Sum2/1
  Product1/1 -> Sum2/2
  i_cf_d/1 -> 1/C_gfm/1
  i_cf_q/1 -> "1/C_gfm "/1

== system subsystem_118_bus_self_clearing_blocking/Subsystem1/area1/ibr/gfm/p measurement delay ==
  in : Inport
  Integrator1 : Integrator  InitialCondition=Subsystem.gfm.p_ref  ContinuousStateAttributes='gfm_p_m'
  Sum2 : Sum  Inputs=-+
  p_meas_bw : Gain  Gain=Subsystem.gfm.p_meas_w
  out : Outport
  wires:
  in/1 -> Sum2/2
  Sum2/1 -> p_meas_bw/1
  Integrator1/1 -> Sum2/1, out/1
  p_meas_bw/1 -> Integrator1/1

== system subsystem_118_bus_self_clearing_blocking/Subsystem1/area1/ibr/gfm/q measurement delay ==
  in : Inport
  Integrator1 : Integrator  InitialCondition=Subsystem.gfm.q_ref  ContinuousStateAttributes='gfm_q_m'
  Sum2 : Sum  Inputs=-+
  p_meas_bw : Gain  Gain=Subsystem.gfm.p_meas_w
  out : Outport
  wires:
  p_meas_bw/1 -> Integrator1/1
  Integrator1/1 -> out/1, Sum2/1
  Sum2/1 -> p_meas_bw/1
  in/1 -> Sum2/2

== system subsystem_118_bus_self_clearing_blocking/Subsystem1/area1/ibr/gfm/simplified current loop d-axis ==
  " " : Inport
  Display : Display
  Gain : Gain  Gain=Subsystem.gfm.i_loop_w
  Integrator1 : Integrator  InitialCondition=Subsystem.gfm.i_d  ContinuousStateAttributes='gfm_id_ctrl'
  Sum2 : Sum  Inputs=-+
  "  " : Outport
  wires:
  Gain/1 -> Display/1, Integrator1/1
  Integrator1/1 -> "  "/1, Sum2/1
  Sum2/1 -> Gain/1
  " "/1 -> Sum2/2

== system subsystem_118_bus_self_clearing_blocking/Subsystem1/area1/ibr/gfm/simplified current loop q-axis ==
  " " : Inport
  Gain : Gain  Gain=Subsystem.gfm.i_loop_w
  Integrator1 : Integrator  InitialCondition=Subsystem.gfm.i_q  ContinuousStateAttributes='gfm_iq_ctrl'
  Sum2 : Sum  Inputs=-+
  "  " : Outport
  wires:
  " "/1 -> Sum2/2
  Sum2/1 -> Gain/1
  Integrator1/1 -> Sum2/1, "  "/1
  Gain/1 -> Integrator1/1

== system subsystem_118_bus_self_clearing_blocking/Subsystem1/area1/ibr/gfm/v measurement delay ==
  in : Inport
  Integrator1 : Integrator  InitialCondition=Subsystem.gfm.v_ref  ContinuousStateAttributes='gfm_v_m'
  Sum2 : Sum  Inputs=-+
  v_meas_bw : Gain  Gain=Subsystem.gfm.q_meas_w
  out : Outport
  wires:
  v_meas_bw/1 -> Integrator1/1
  Integrator1/1 -> out/1, Sum2/1
  Sum2/1 -> v_meas_bw/1
  in/1 -> Sum2/2

== system subsystem_118_bus_self_clearing_blocking/Subsystem1/area1/ibr/gfm/vd_loop_pi ==
  "  " : Inport
  Integrator : Integrator  ContinuousStateAttributes='gfm_vd_ctrl'
  Ki : Gain  Gain=Subsystem.gfm_gains.vd_ki
  Kp : Gain  Gain=Subsystem.gfm_gains.vd_kp
  Sum : Sum  Inputs=|++
  " " : Outport
  wires:
  Kp/1 -> Sum/1
  Integrator/1 -> Sum/2
  Ki/1 -> Integrator/1
  "  "/1 -> Ki/1, Kp/1
  Sum/1 -> " "/1

== system subsystem_118_bus_self_clearing_blocking/Subsystem1/area1/ibr/gfm/vq_loop_pi ==
  "  " : Inport
  Integrator : Integrator  ContinuousStateAttributes='gfm_vq_ctrl'
  Ki : Gain  Gain=Subsystem.gfm_gains.vq_ki
  Kp : Gain  Gain=Subsystem.gfm_gains.vq_kp
  Sum : Sum  Inputs=|++
  " " : Outport
  wires:
  Sum/1 -> " "/1
  "  "/1 -> Kp/1, Ki/1
  Ki/1 -> Integrator/1
  Integrator/1 -> Sum/2
  Kp/1 -> Sum/1

== system subsystem_118_bus_self_clearing_blocking/Subsystem1/area1/non_ibr/floating buses/line charging dynamics ==
  note: I am multiplying here by negative
  note: I am multiplying here by negative
  i_float_D : Inport
  i_float_Q : Inport  Port=2
  " " : Integrator  InitialCondition=Subsystem.float.v_D  ContinuousStateAttributes='floatvD'
  1/C_float : Gain  Gain=-1./Subsystem.float.c
  "1/C_float " : Gain  Gain=-1./Subsystem.float.c
  Constant : Constant  Value=w
  Integrator1 : Integrator  InitialCondition=Subsystem.float.v_Q  ContinuousStateAttributes='floatvQ'
  Product : Product
  Product1 : Product
  Sum2 : Sum  Inputs=+-
  Sum3 : Sum
  v_float_D : Outport
  v_float_Q : Outport  Port=2
  wires:
  " "/1 -> Product1/1, v_float_D/1
  Integrator1/1 -> v_float_Q/1, Product/2
  [ws] -> Product1/2
  Sum3/1 -> " "/1
  Sum2/1 -> Integrator1/1
  1/C_float/1 -> Sum3/2
  Product/1 -> Sum3/1
  "1/C_float "/1 -> Sum2/1
  Product1/1 -> Sum2/2
  i_float_D/1 -> 1/C_float/1
  i_float_Q/1 -> "1/C_float "/1
  [ws] -> Product/1
  Constant/1 -> [ws]

== system subsystem_118_bus_self_clearing_blocking/Subsystem1/area1/non_ibr/load buses/Subsystem ==
  p : Inport
  q : Inport  Port=2
  vD : Inport  Port=3
  vQ : Inport  Port=4
  Complex to Real-Imag : ComplexToRealImag
  Conj : Math  Operator=conj
  Divide : Product  Inputs=*/
  Real-Imag to Complex : RealImagToComplex
  Real-Imag to Complex1 : RealImagToComplex
  i_inj_load_d : Outport
  i_inj_load_q : Outport  Port=2
  wires:
  q/1 -> Real-Imag to Complex/2
  Real-Imag to Complex1/1 -> Divide/2
  Divide/1 -> Conj/1
  Complex to Real-Imag/2 -> i_inj_load_q/1
  Real-Imag to Complex/1 -> Divide/1
  vQ/1 -> Real-Imag to Complex1/2
  vD/1 -> Real-Imag to Complex1/1
  Complex to Real-Imag/1 -> i_inj_load_d/1
  p/1 -> Real-Imag to Complex/1
  Conj/1 -> Complex to Real-Imag/1

== system subsystem_118_bus_self_clearing_blocking/Subsystem1/area1/non_ibr/load buses/line charging dynamics ==
  i_load_c_D : Inport
  i_load_c_Q : Inport  Port=2
  " " : Integrator  InitialCondition=Subsystem.load1.v_D  ContinuousStateAttributes='loadvD'
  1/C_load : Gain  Gain=1./Subsystem.load1.c
  "1/C_load " : Gain  Gain=1./Subsystem.load1.c
  Constant : Constant  Value=w
  Integrator1 : Integrator  InitialCondition=Subsystem.load1.v_Q  ContinuousStateAttributes='loadvQ'
  Product : Product
  Product1 : Product
  Sum2 : Sum  Inputs=+-
  Sum3 : Sum
  v_load_D : Outport
  v_load_Q : Outport  Port=2
  wires:
  [ws] -> Product/1
  " "/1 -> Product1/1, v_load_D/1
  Integrator1/1 -> v_load_Q/1, Product/2
  [ws] -> Product1/2
  Sum3/1 -> " "/1
  Sum2/1 -> Integrator1/1
  1/C_load/1 -> Sum3/2
  Product/1 -> Sum3/1
  "1/C_load "/1 -> Sum2/1
  Product1/1 -> Sum2/2
  i_load_c_D/1 -> 1/C_load/1
  i_load_c_Q/1 -> "1/C_load "/1
  Constant/1 -> [ws]

== system subsystem_118_bus_self_clearing_blocking/Subsystem2/area2/ibr/gfl/DQ//dq ==
  D_quantity : Inport
  Q_quantity : Inport  Port=2
  theta : Inport  Port=3
  Complex to Magnitude-Angle : ComplexToMagnitudeAngle
  Complex to Real-Imag : ComplexToRealImag
  Magnitude-Angle to Complex : MagnitudeAngleToComplex
  Real-Imag to Complex : RealImagToComplex
  Sum : Sum  Inputs=|+-
  d_quantity : Outport
  q_quantity : Outport  Port=2
  wires:
  D_quantity/1 -> Real-Imag to Complex/1
  Complex to Magnitude-Angle/2 -> Sum/1
  Complex to Magnitude-Angle/1 -> Magnitude-Angle to Complex/1
  Real-Imag to Complex/1 -> Complex to Magnitude-Angle/1
  Sum/1 -> Magnitude-Angle to Complex/2
  Q_quantity/1 -> Real-Imag to Complex/2
  Magnitude-Angle to Complex/1 -> Complex to Real-Imag/1
  Complex to Real-Imag/1 -> d_quantity/1
  Complex to Real-Imag/2 -> q_quantity/1
  theta/1 -> Sum/2

== system subsystem_118_bus_self_clearing_blocking/Subsystem2/area2/ibr/gfl/Subsystem ==
  vbDQ : Inport
  Abs : Abs  SaturateOnIntegerOverflow=off
  Vm : Outport
  wires:
  Abs/1 -> Vm/1
  vbDQ/1 -> Abs/1

== system subsystem_118_bus_self_clearing_blocking/Subsystem2/area2/ibr/gfl/Subsystem1 ==
  vbDQ : Inport
  IbDQ : Inport  Port=2
  Complex to Real-Imag : ComplexToRealImag
  Complex to Real-Imag1 : ComplexToRealImag
  Product{,1..3} (4 alike) : Product
  Sum : Sum
  Sum1 : Sum  Inputs=+-
  Pm : Outport
  Qm : Outport  Port=2
  wires:
  Product/1 -> Sum/1
  Product1/1 -> Sum/2
  Sum/1 -> Pm/1
  Sum1/1 -> Qm/1
  Product3/1 -> Sum1/2
  Product2/1 -> Sum1/1
  [vbQ] -> Product2/1
  [IbD] -> Product2/2
  [vbD] -> Product3/1
  [IbQ] -> Product3/2
  [vbD] -> Product/1
  [IbD] -> Product/2
  [IbQ] -> Product1/2
  [vbQ] -> Product1/1
  vbDQ/1 -> Complex to Real-Imag/1
  Complex to Real-Imag/1 -> [vbD]
  Complex to Real-Imag/2 -> [vbQ]
  IbDQ/1 -> Complex to Real-Imag1/1
  Complex to Real-Imag1/1 -> [IbD]
  Complex to Real-Imag1/2 -> [IbQ]

== system subsystem_118_bus_self_clearing_blocking/Subsystem2/area2/ibr/gfl/dq//DQ ==
  d-quantity : Inport
  q-quantity : Inport  Port=2
  theta : Inport  Port=3
  Complex to Magnitude-Angle : ComplexToMagnitudeAngle
  Complex to Real-Imag : ComplexToRealImag
  Magnitude-Angle to Complex : MagnitudeAngleToComplex
  Real-Imag to Complex : RealImagToComplex
  Sum : Sum  Inputs=|++
  D-quantity : Outport
  Q-quantity : Outport  Port=2
  wires:
  d-quantity/1 -> Real-Imag to Complex/1
  Complex to Magnitude-Angle/2 -> Sum/1
  Complex to Magnitude-Angle/1 -> Magnitude-Angle to Complex/1
  Real-Imag to Complex/1 -> Complex to Magnitude-Angle/1
  Sum/1 -> Magnitude-Angle to Complex/2
  q-quantity/1 -> Real-Imag to Complex/2
  Magnitude-Angle to Complex/1 -> Complex to Real-Imag/1
  Complex to Real-Imag/1 -> D-quantity/1
  Complex to Real-Imag/2 -> Q-quantity/1
  theta/1 -> Sum/2

== system subsystem_118_bus_self_clearing_blocking/Subsystem2/area2/ibr/gfl/filter capacitor dynamics ==
  i_cf_d : Inport
  w : Inport  Port=2
  i_cf_q : Inport  Port=3
  1/C_gfl_pv : Gain  Gain=1./Subsystem.gfl.c
  "1/C_gfl_pv " : Gain  Gain=1./Subsystem.gfl.c
  Integrator : Integrator  InitialCondition=Subsystem.gfl.v_d  ContinuousStateAttributes='gfl_vd'
  Integrator1 : Integrator  InitialCondition=Subsystem.gfl.v_q  ContinuousStateAttributes='gfl_vq'
  Product : Product
  Product1 : Product
  Sum2 : Sum  Inputs=+-
  Sum3 : Sum
  v_gfl_d : Outport
  v_gfl_q : Outport  Port=2
  wires:
  w/1 -> [ws]
  [ws] -> Product/1
  Integrator/1 -> Product1/1, v_gfl_d/1
  Integrator1/1 -> Product/2, v_gfl_q/1
  [ws] -> Product1/2
  Sum3/1 -> Integrator/1
  Sum2/1 -> Integrator1/1
  1/C_gfl_pv/1 -> Sum3/2
  Product/1 -> Sum3/1
  "1/C_gfl_pv "/1 -> Sum2/1
  Product1/1 -> Sum2/2
  i_cf_d/1 -> 1/C_gfl_pv/1
  i_cf_q/1 -> "1/C_gfl_pv "/1

== system subsystem_118_bus_self_clearing_blocking/Subsystem2/area2/ibr/gfl/p measurement delay ==
  in : Inport
  Integrator1 : Integrator  InitialCondition=Subsystem.gfl.p_ref  ContinuousStateAttributes='gfl_p_m'
  Sum2 : Sum  Inputs=-+
  p_meas_bw : Gain  Gain=Subsystem.gfl.p_meas_w
  out : Outport
  wires:
  in/1 -> Sum2/2
  Sum2/1 -> p_meas_bw/1
  Integrator1/1 -> Sum2/1, out/1
  p_meas_bw/1 -> Integrator1/1

== system subsystem_118_bus_self_clearing_blocking/Subsystem2/area2/ibr/gfl/p_loop_pi ==
  "  " : Inport
  Integrator : Integrator  ContinuousStateAttributes='gfl_p_ctrl'
  Ki : Gain  Gain=Subsystem.gfl_gains.kip
  Kp : Gain  Gain=Subsystem.gfl_gains.kpp
  Sum : Sum  Inputs=|++
  " " : Outport
  wires:
  Kp/1 -> Sum/1
  Integrator/1 -> Sum/2
  Ki/1 -> Integrator/1
  "  "/1 -> Ki/1, Kp/1
  Sum/1 -> " "/1

== system subsystem_118_bus_self_clearing_blocking/Subsystem2/area2/ibr/gfl/pll_lpf ==
  LPF_input : Inport
  Integrator1 : Integrator  ContinuousStateAttributes='gfl_pll_lpf'
  Sum2 : Sum  Inputs=-+
  pll_lpf_bw : Gain  Gain=Subsystem.gfl.pll_lpf_w
  LPF_output : Outport
  wires:
  pll_lpf_bw/1 -> Integrator1/1
  Integrator1/1 -> LPF_output/1, Sum2/1
  Sum2/1 -> pll_lpf_bw/1
  LPF_input/1 -> Sum2/2

== system subsystem_118_bus_self_clearing_blocking/Subsystem2/area2/ibr/gfl/pll_pi ==
  "  " : Inport
  Integrator : Integrator  ContinuousStateAttributes='gfl_pll'
  Ki : Gain  Gain=Subsystem.gfl_gains.kipll
  Kp : Gain  Gain=Subsystem.gfl_gains.kppll
  Sum : Sum  Inputs=|++
  " " : Outport
  wires:
  Kp/1 -> Sum/1
  Integrator/1 -> Sum/2
  Ki/1 -> Integrator/1
  "  "/1 -> Ki/1, Kp/1
  Sum/1 -> " "/1

== system subsystem_118_bus_self_clearing_blocking/Subsystem2/area2/ibr/gfl/simplified current loop d-axis ==
  " " : Inport
  Gain : Gain  Gain=Subsystem.gfl.i_loop_w
  Integrator1 : Integrator  InitialCondition=Subsystem.gfl.i_d  ContinuousStateAttributes='gfl_id_ctrl'
  Sum2 : Sum  Inputs=-+
  "  " : Outport
  wires:
  Gain/1 -> Integrator1/1
  Integrator1/1 -> "  "/1, Sum2/1
  Sum2/1 -> Gain/1
  " "/1 -> Sum2/2

== system subsystem_118_bus_self_clearing_blocking/Subsystem2/area2/ibr/gfl/simplified current loop q-axis ==
  i_gfl_q : Inport
  Gain : Gain  Gain=Subsystem.gfl.i_loop_w
  Integrator1 : Integrator  InitialCondition=Subsystem.gfl.i_q  ContinuousStateAttributes='gfl_iq_ctrl'
  Sum2 : Sum  Inputs=-+
  igfl_q : Outport
  wires:
  Gain/1 -> Integrator1/1
  Integrator1/1 -> igfl_q/1, Sum2/1
  Sum2/1 -> Gain/1
  i_gfl_q/1 -> Sum2/2

== system subsystem_118_bus_self_clearing_blocking/Subsystem2/area2/ibr/gfl/v measurement delay ==
  in : Inport
  Integrator1 : Integrator  InitialCondition=Subsystem.gfl.v_ref  ContinuousStateAttributes='gfl_v_m'
  Sum2 : Sum  Inputs=-+
  v_meas_bw : Gain  Gain=Subsystem.gfl.v_meas_w
  out : Outport
  wires:
  in/1 -> Sum2/2
  Sum2/1 -> v_meas_bw/1
  Integrator1/1 -> Sum2/1, out/1
  v_meas_bw/1 -> Integrator1/1

== system subsystem_118_bus_self_clearing_blocking/Subsystem2/area2/ibr/gfl/v_loop_pi ==
  "  " : Inport
  Integrator : Integrator  ContinuousStateAttributes='gfl_v_ctrl'
  Ki : Gain  Gain=Subsystem.gfl_gains.kiv
  Kp : Gain  Gain=Subsystem.gfl_gains.kpv
  Sum : Sum  Inputs=|++
  " " : Outport
  wires:
  Kp/1 -> Sum/1
  Integrator/1 -> Sum/2
  Ki/1 -> Integrator/1
  "  "/1 -> Ki/1, Kp/1
  Sum/1 -> " "/1
